simulink model "corner_detection_2019b"  (Simulink 10.0)
settings: Solver=FixedStepDiscrete  StartTime=0.0  StopTime=0  RelTol=1e-3  EnableMultiTasking=on
undefined symbols (not defined in the file or in its folder): fspecial, gray, Rec, SDTV
libraries: visionconversions x1, visionanalysis x1, visiontextngfix x1, visionsources x1
settings Model: Creator=FxMain  LastModifiedBy=panos  PacingRate=0.001800
settings DataIOCC: LimitDataPoints=on
settings OptimizationCC: ExpressionDepthLimit=2147483647
settings DebuggingCC: SolverPrmCheckMsg=warning  FcnCallInpInsideContextMsg=warning  StateNameClashWarn=warning
settings ConfigComp: CovExternalEMLEnable=off

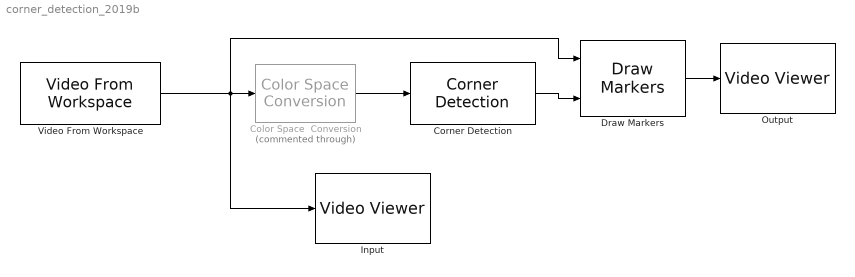
== system corner_detection_2019b ==
  Color Space  Conversion : visionconversions/Color Space  Conversion  Commented=through  conversion=Obsolete  conversionActive=R'G'B' to intensity  wp_str=D65  rec=Rec. 601 (SDTV)  sys=1125/60/2:1  imagePorts=One multidimensional signal
  Corner Detection : visionanalysis/Corner Detection  method=Local intensity comparison (Rosen & Drummond)  factor=0.04  filter=fspecial('gaussian', [1 5], 1.5)  thrInten=0.1  thrAngle=157.5  output=Obsolete9b  outputInUse=Corner location  maxNum=20  thrMetric=0.0005  neighborSize=[5 5]  isOutVarDim=on  roundingMode=Floor  overflowMode=off  firstCoeffMode=Specify word length  firstCoeffWordLength=16  firstCoeffFracLength=16  prodOutputMode=Binary point scaling  prodOutputWordLength=32  prodOutputFracLength=0  accumMode=Binary point scaling  accumWordLength=32  accumFracLength=0  memoryMode=Binary point scaling  memoryWordLength=32  memoryFracLength=0
      settings: SourceProductBaseCode=VP
  Draw Markers : visiontextngfix/Draw Markers  shape=Circle  size=20  fill=on  fillClrSource=Specify via dialog  display=White  intensity=200  color=255  opacity=0.6  viewport=Entire image  antialiasing=off  inType=Obsolete  imagePorts=One multidimensional signal  roundingMode=Floor  overflowMode=off  memoryMode=Specify word length  memoryWordLength=16  memoryFracLength=15  prodOutputMode=Binary point scaling  prodOutputWordLength=32  prodOutputFracLength=14
      settings: SourceProductBaseCode=VP
  Input : VideoViewer  colormapValue=gray(256)  FigPos=[2290 910 992 635]
  Output : VideoViewer  colormapValue=gray(256)  FigPos=[2498 941 1228 608]
  Video From Workspace : visionsources/Video From Workspace  signal=vid1  Ts=1  finalout=Obsolete  finaloutActive=Cyclic repetition  imagePorts=One multidimensional signal  OutPortLabels=R|G|B
      settings: SourceProductBaseCode=VP
  wires:
  Video From Workspace/1 -> Input/1, Draw Markers/1, Color Space  Conversion/1
  Color Space  Conversion/1 -> Corner Detection/1
  Corner Detection/1 -> Draw Markers/2
  Draw Markers/1 -> Output/1
